simulink model "TST_TCPrt_TrqLim"  (R2016b)
settings: Solver=FixedStepDiscrete  StartTime=0.0  StopTime=simTime  FixedStep=sampleTime  RelTol=1e-3
values from neighbouring files (symbols this model uses):
  testCase = 1    [initTST_TCPrt_TrqLim_001.m]    (also in initTST_TCPrt_TrqLim_002.m = 2)
libraries: simulink x3
settings Model: Creator=wolf072601  LastModifiedBy=wolf072601
settings DebuggingCC: SignalRangeChecking=error

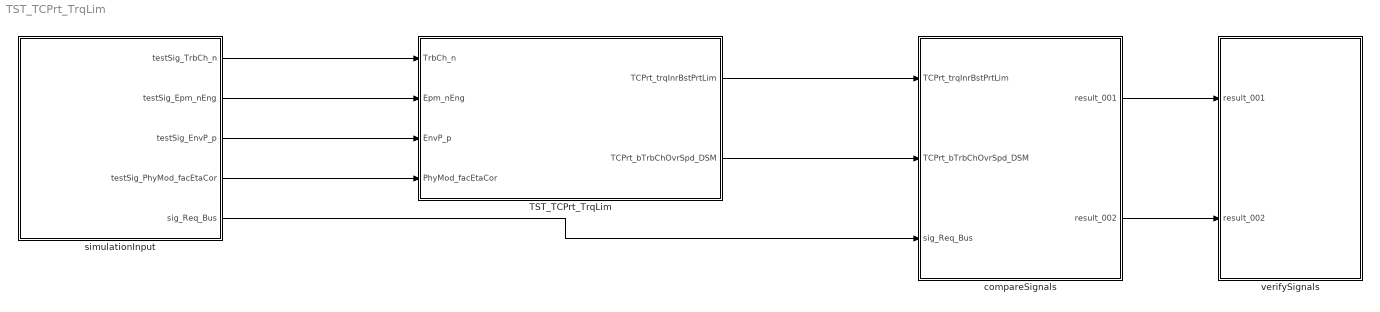
== system TST_TCPrt_TrqLim ==
  TST_TCPrt_TrqLim : Subsystem
  compareSignals : Subsystem
  simulationInput : Subsystem
  verifySignals : Subsystem
  wires:
  simulationInput/1(testSig_TrbCh_n) -> TST_TCPrt_TrqLim/1(TrbCh_n)
  simulationInput/2(testSig_Epm_nEng) -> TST_TCPrt_TrqLim/2(Epm_nEng)
  simulationInput/3(testSig_EnvP_p) -> TST_TCPrt_TrqLim/3(EnvP_p)
  simulationInput/4(testSig_PhyMod_facEtaCor) -> TST_TCPrt_TrqLim/4(PhyMod_facEtaCor)
  TST_TCPrt_TrqLim/1(TCPrt_trqInrBstPrtLim) -> compareSignals/1(TCPrt_trqInrBstPrtLim)
  TST_TCPrt_TrqLim/2(TCPrt_bTrbChOvrSpd_DSM) -> compareSignals/2(TCPrt_bTrbChOvrSpd_DSM)
  simulationInput/5(sig_Req_Bus) -> compareSignals/3(sig_Req_Bus)
  compareSignals/1(result_001) -> verifySignals/1(result_001)
  compareSignals/2(result_002) -> verifySignals/2(result_002)

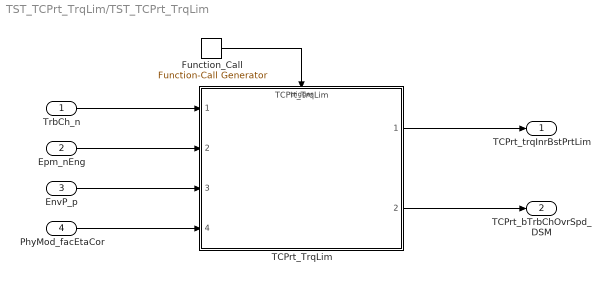
== system TST_TCPrt_TrqLim/TST_TCPrt_TrqLim ==
  TrbCh_n : Inport
  Epm_nEng : Inport  Port=2
  EnvP_p : Inport  Port=3
  PhyMod_facEtaCor : Inport  Port=4
  Function_Call : simulink/Ports & Subsystems/Function-Call Generator  sample_time=sampleTime  numberOfIterations=1
  TCPrt_TrqLim : ModelReference  ModelNameDialog=TCPrt_TrqLim  ModelReferenceVersion=1.14  TriggerPortName=function  TriggerPortTriggerType=function-call  TriggerPortStatesWhenEnabling=held
  TCPrt_trqInrBstPrtLim : Outport
  TCPrt_bTrbChOvrSpd_DSM : Outport  Port=2
  wires:
  Function_Call/1 -> TCPrt_TrqLim/Trigger
  TrbCh_n/1 -> TCPrt_TrqLim/1
  Epm_nEng/1 -> TCPrt_TrqLim/2
  EnvP_p/1 -> TCPrt_TrqLim/3
  PhyMod_facEtaCor/1 -> TCPrt_TrqLim/4
  TCPrt_TrqLim/1 -> TCPrt_trqInrBstPrtLim/1
  TCPrt_TrqLim/2 -> TCPrt_bTrbChOvrSpd_DSM/1

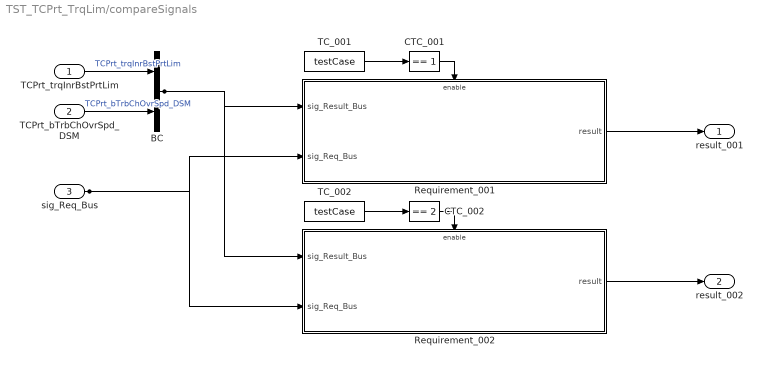
== system TST_TCPrt_TrqLim/compareSignals ==
  TCPrt_trqInrBstPrtLim : Inport
  TCPrt_bTrbChOvrSpd_DSM : Inport  Port=2
  sig_Req_Bus : Inport  Port=3
  BC : BusCreator  Inputs=2
  CTC_001 : simulink/Logic and Bit Operations/Compare To Constant  relop===  const=1  OutDataTypeStr=boolean
  CTC_002 : simulink/Logic and Bit Operations/Compare To Constant  relop===  const=2  OutDataTypeStr=boolean
  Requirement_001 : Subsystem
  Requirement_002 : Subsystem
  TC_001 : Constant  Value=testCase
  TC_002 : Constant  Value=testCase
  result_001 : Outport
  result_002 : Outport  Port=2
  wires:
  TCPrt_trqInrBstPrtLim/1 -> BC/1  "TCPrt_trqInrBstPrtLim"
  TCPrt_bTrbChOvrSpd_DSM/1 -> BC/2  "TCPrt_bTrbChOvrSpd_DSM"
  TC_001/1 -> CTC_001/1
  CTC_001/1 -> Requirement_001/Enable
  sig_Req_Bus/1 -> Requirement_001/2(sig_Req_Bus), Requirement_002/2(sig_Req_Bus)
  BC/1 -> Requirement_001/1(sig_Result_Bus), Requirement_002/1(sig_Result_Bus)
  Requirement_001/1(result) -> result_001/1
  TC_002/1 -> CTC_002/1
  CTC_002/1 -> Requirement_002/Enable
  Requirement_002/1(result) -> result_002/1

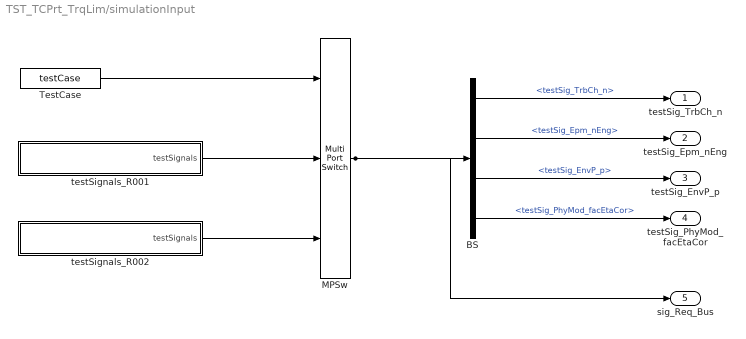
== system TST_TCPrt_TrqLim/simulationInput ==
  BS : BusSelector  OutputSignals=testSig_TrbCh_n,testSig_Epm_nEng,testSig_EnvP_p,testSig_PhyMod_facEtaCor
  MPSw : MultiPortSwitch  Inputs=2  SaturateOnIntegerOverflow=on  InputSameDT=on
  TestCase : Constant  Value=testCase
  testSignals_R001 : Subsystem
  testSignals_R002 : Subsystem
  testSig_TrbCh_n : Outport
  testSig_Epm_nEng : Outport  Port=2
  testSig_EnvP_p : Outport  Port=3
  testSig_PhyMod_facEtaCor : Outport  Port=4
  sig_Req_Bus : Outport  Port=5
  wires:
  BS/1 -> testSig_TrbCh_n/1  "<testSig_TrbCh_n>"
  BS/2 -> testSig_Epm_nEng/1  "<testSig_Epm_nEng>"
  BS/3 -> testSig_EnvP_p/1  "<testSig_EnvP_p>"
  BS/4 -> testSig_PhyMod_facEtaCor/1  "<testSig_PhyMod_facEtaCor>"
  MPSw/1 -> BS/1, sig_Req_Bus/1
  TestCase/1 -> MPSw/1
  testSignals_R001/1(testSignals) -> MPSw/2
  testSignals_R002/1(testSignals) -> MPSw/3

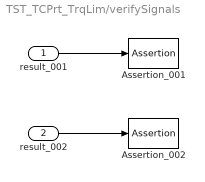
== system TST_TCPrt_TrqLim/verifySignals ==
  result_001 : Inport
  result_002 : Inport  Port=2
  Assertion_001 : Assertion  Enabled=off
  Assertion_002 : Assertion  Enabled=off
  wires:
  result_001/1 -> Assertion_001/1
  result_002/1 -> Assertion_002/1

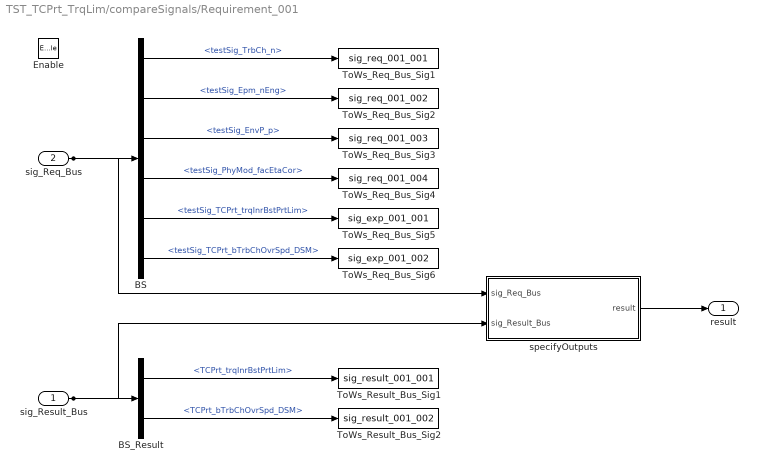
== system TST_TCPrt_TrqLim/compareSignals/Requirement_001 ==
  sig_Result_Bus : Inport
  sig_Req_Bus : Inport  Port=2
  Enable : EnablePort
  BS : BusSelector  OutputSignals=testSig_TrbCh_n,testSig_Epm_nEng,testSig_EnvP_p,testSig_PhyMod_facEtaCor,testSig_TCPrt_trqInrBstPrtLim,testSig_TCPrt_bTrbChOvrSpd_DSM
  BS_Result : BusSelector  OutputSignals=TCPrt_trqInrBstPrtLim,TCPrt_bTrbChOvrSpd_DSM
  ToWs_Req_Bus_Sig1 : ToWorkspace  VariableName=sig_req_001_001  SaveFormat=Structure With Time
  ToWs_Req_Bus_Sig2 : ToWorkspace  VariableName=sig_req_001_002  SaveFormat=Structure With Time
  ToWs_Req_Bus_Sig3 : ToWorkspace  VariableName=sig_req_001_003  SaveFormat=Structure With Time
  ToWs_Req_Bus_Sig4 : ToWorkspace  VariableName=sig_req_001_004  SaveFormat=Structure With Time
  ToWs_Req_Bus_Sig5 : ToWorkspace  VariableName=sig_exp_001_001  SaveFormat=Structure With Time
  ToWs_Req_Bus_Sig6 : ToWorkspace  VariableName=sig_exp_001_002  SaveFormat=Structure With Time
  ToWs_Result_Bus_Sig1 : ToWorkspace  VariableName=sig_result_001_001  SaveFormat=Structure With Time
  ToWs_Result_Bus_Sig2 : ToWorkspace  VariableName=sig_result_001_002  SaveFormat=Structure With Time
  specifyOutputs : Subsystem
  result : Outport
  wires:
  sig_Req_Bus/1 -> BS/1, specifyOutputs/1(sig_Req_Bus)
  BS/1 -> ToWs_Req_Bus_Sig1/1  "<testSig_TrbCh_n>"
  BS/2 -> ToWs_Req_Bus_Sig2/1  "<testSig_Epm_nEng>"
  BS/3 -> ToWs_Req_Bus_Sig3/1  "<testSig_EnvP_p>"
  BS/4 -> ToWs_Req_Bus_Sig4/1  "<testSig_PhyMod_facEtaCor>"
  BS/5 -> ToWs_Req_Bus_Sig5/1  "<testSig_TCPrt_trqInrBstPrtLim>"
  BS/6 -> ToWs_Req_Bus_Sig6/1  "<testSig_TCPrt_bTrbChOvrSpd_DSM>"
  sig_Result_Bus/1 -> BS_Result/1, specifyOutputs/2(sig_Result_Bus)
  BS_Result/1 -> ToWs_Result_Bus_Sig1/1  "<TCPrt_trqInrBstPrtLim>"
  BS_Result/2 -> ToWs_Result_Bus_Sig2/1  "<TCPrt_bTrbChOvrSpd_DSM>"
  specifyOutputs/1(result) -> result/1

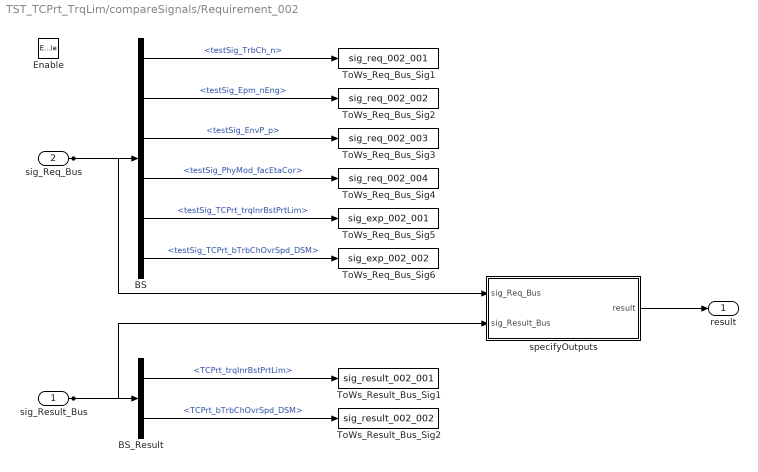
== system TST_TCPrt_TrqLim/compareSignals/Requirement_002 ==
  sig_Result_Bus : Inport
  sig_Req_Bus : Inport  Port=2
  Enable : EnablePort
  BS : BusSelector  OutputSignals=testSig_TrbCh_n,testSig_Epm_nEng,testSig_EnvP_p,testSig_PhyMod_facEtaCor,testSig_TCPrt_trqInrBstPrtLim,testSig_TCPrt_bTrbChOvrSpd_DSM
  BS_Result : BusSelector  OutputSignals=TCPrt_trqInrBstPrtLim,TCPrt_bTrbChOvrSpd_DSM
  ToWs_Req_Bus_Sig1 : ToWorkspace  VariableName=sig_req_002_001  SaveFormat=Structure With Time
  ToWs_Req_Bus_Sig2 : ToWorkspace  VariableName=sig_req_002_002  SaveFormat=Structure With Time
  ToWs_Req_Bus_Sig3 : ToWorkspace  VariableName=sig_req_002_003  SaveFormat=Structure With Time
  ToWs_Req_Bus_Sig4 : ToWorkspace  VariableName=sig_req_002_004  SaveFormat=Structure With Time
  ToWs_Req_Bus_Sig5 : ToWorkspace  VariableName=sig_exp_002_001  SaveFormat=Structure With Time
  ToWs_Req_Bus_Sig6 : ToWorkspace  VariableName=sig_exp_002_002  SaveFormat=Structure With Time
  ToWs_Result_Bus_Sig1 : ToWorkspace  VariableName=sig_result_002_001  SaveFormat=Structure With Time
  ToWs_Result_Bus_Sig2 : ToWorkspace  VariableName=sig_result_002_002  SaveFormat=Structure With Time
  specifyOutputs : Subsystem
  result : Outport
  wires:
  sig_Req_Bus/1 -> BS/1, specifyOutputs/1(sig_Req_Bus)
  BS/1 -> ToWs_Req_Bus_Sig1/1  "<testSig_TrbCh_n>"
  BS/2 -> ToWs_Req_Bus_Sig2/1  "<testSig_Epm_nEng>"
  BS/3 -> ToWs_Req_Bus_Sig3/1  "<testSig_EnvP_p>"
  BS/4 -> ToWs_Req_Bus_Sig4/1  "<testSig_PhyMod_facEtaCor>"
  BS/5 -> ToWs_Req_Bus_Sig5/1  "<testSig_TCPrt_trqInrBstPrtLim>"
  BS/6 -> ToWs_Req_Bus_Sig6/1  "<testSig_TCPrt_bTrbChOvrSpd_DSM>"
  sig_Result_Bus/1 -> BS_Result/1, specifyOutputs/2(sig_Result_Bus)
  BS_Result/1 -> ToWs_Result_Bus_Sig1/1  "<TCPrt_trqInrBstPrtLim>"
  BS_Result/2 -> ToWs_Result_Bus_Sig2/1  "<TCPrt_bTrbChOvrSpd_DSM>"
  specifyOutputs/1(result) -> result/1

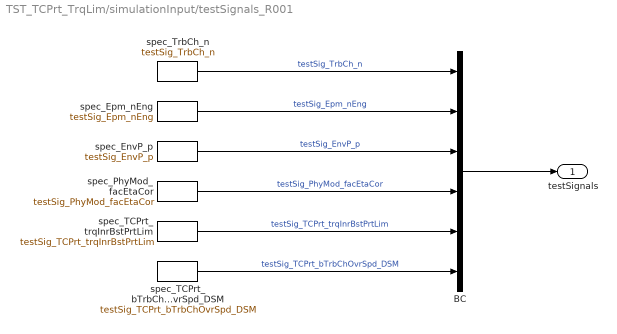
== system TST_TCPrt_TrqLim/simulationInput/testSignals_R001 ==
  BC : BusCreator  Inputs=6
  spec_EnvP_p : FromWorkspace  VariableName=testSig_EnvP_p  Interpolate=off  OutputAfterFinalValue=Holding final value
  spec_Epm_nEng : FromWorkspace  VariableName=testSig_Epm_nEng  Interpolate=off  OutputAfterFinalValue=Holding final value
  spec_PhyMod_facEtaCor : FromWorkspace  VariableName=testSig_PhyMod_facEtaCor  Interpolate=off  OutputAfterFinalValue=Holding final value
  spec_TCPrt_bTrbChOvrSpd_DSM : FromWorkspace  VariableName=testSig_TCPrt_bTrbChOvrSpd_DSM  Interpolate=off  OutputAfterFinalValue=Holding final value
  spec_TCPrt_trqInrBstPrtLim : FromWorkspace  VariableName=testSig_TCPrt_trqInrBstPrtLim  Interpolate=off  OutputAfterFinalValue=Holding final value
  spec_TrbCh_n : FromWorkspace  VariableName=testSig_TrbCh_n  Interpolate=off  OutputAfterFinalValue=Holding final value
  testSignals : Outport
  wires:
  BC/1 -> testSignals/1
  spec_TrbCh_n/1 -> BC/1  "testSig_TrbCh_n"
  spec_Epm_nEng/1 -> BC/2  "testSig_Epm_nEng"
  spec_EnvP_p/1 -> BC/3  "testSig_EnvP_p"
  spec_PhyMod_facEtaCor/1 -> BC/4  "testSig_PhyMod_facEtaCor"
  spec_TCPrt_trqInrBstPrtLim/1 -> BC/5  "testSig_TCPrt_trqInrBstPrtLim"
  spec_TCPrt_bTrbChOvrSpd_DSM/1 -> BC/6  "testSig_TCPrt_bTrbChOvrSpd_DSM"

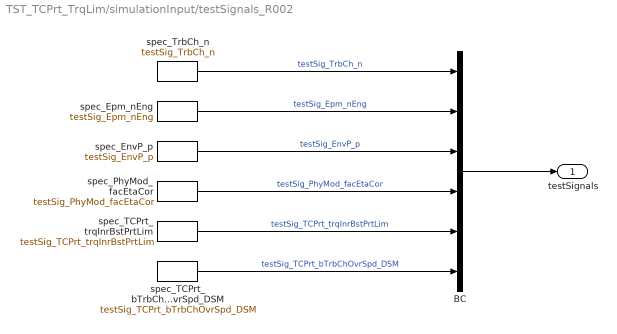
== system TST_TCPrt_TrqLim/simulationInput/testSignals_R002 ==
  BC : BusCreator  Inputs=6
  spec_EnvP_p : FromWorkspace  VariableName=testSig_EnvP_p  Interpolate=off  OutputAfterFinalValue=Holding final value
  spec_Epm_nEng : FromWorkspace  VariableName=testSig_Epm_nEng  Interpolate=off  OutputAfterFinalValue=Holding final value
  spec_PhyMod_facEtaCor : FromWorkspace  VariableName=testSig_PhyMod_facEtaCor  Interpolate=off  OutputAfterFinalValue=Holding final value
  spec_TCPrt_bTrbChOvrSpd_DSM : FromWorkspace  VariableName=testSig_TCPrt_bTrbChOvrSpd_DSM  Interpolate=off  OutputAfterFinalValue=Holding final value
  spec_TCPrt_trqInrBstPrtLim : FromWorkspace  VariableName=testSig_TCPrt_trqInrBstPrtLim  Interpolate=off  OutputAfterFinalValue=Holding final value
  spec_TrbCh_n : FromWorkspace  VariableName=testSig_TrbCh_n  Interpolate=off  OutputAfterFinalValue=Holding final value
  testSignals : Outport
  wires:
  BC/1 -> testSignals/1
  spec_TrbCh_n/1 -> BC/1  "testSig_TrbCh_n"
  spec_Epm_nEng/1 -> BC/2  "testSig_Epm_nEng"
  spec_EnvP_p/1 -> BC/3  "testSig_EnvP_p"
  spec_PhyMod_facEtaCor/1 -> BC/4  "testSig_PhyMod_facEtaCor"
  spec_TCPrt_trqInrBstPrtLim/1 -> BC/5  "testSig_TCPrt_trqInrBstPrtLim"
  spec_TCPrt_bTrbChOvrSpd_DSM/1 -> BC/6  "testSig_TCPrt_bTrbChOvrSpd_DSM"

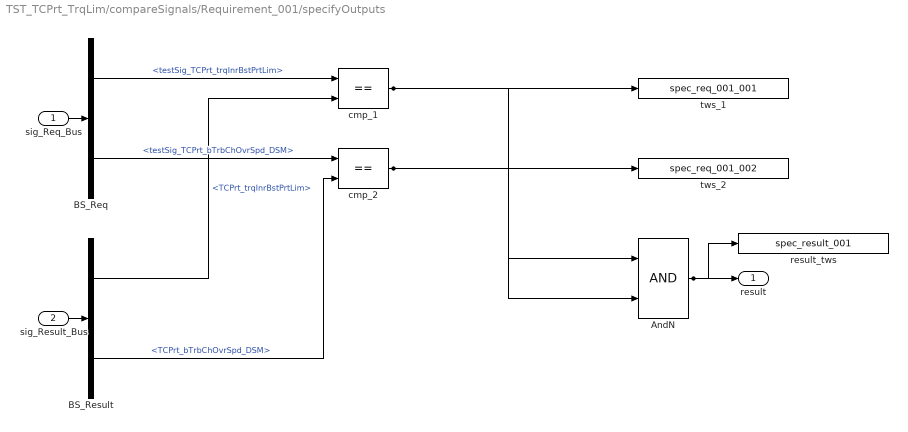
== system TST_TCPrt_TrqLim/compareSignals/Requirement_001/specifyOutputs ==
  sig_Req_Bus : Inport
  sig_Result_Bus : Inport  Port=2
  AndN : Logic
  BS_Req : BusSelector  OutputSignals=testSig_TCPrt_trqInrBstPrtLim,testSig_TCPrt_bTrbChOvrSpd_DSM
  BS_Result : BusSelector  OutputSignals=TCPrt_trqInrBstPrtLim,TCPrt_bTrbChOvrSpd_DSM
  cmp_1 : RelationalOperator  Operator===  RndMeth=Nearest  InputSameDT=on
  cmp_2 : RelationalOperator  Operator===  RndMeth=Nearest  InputSameDT=on
  result_tws : ToWorkspace  VariableName=spec_result_001
  tws_1 : ToWorkspace  VariableName=spec_req_001_001
  tws_2 : ToWorkspace  VariableName=spec_req_001_002
  result : Outport
  wires:
  sig_Req_Bus/1 -> BS_Req/1
  sig_Result_Bus/1 -> BS_Result/1
  AndN/1 -> result/1, result_tws/1
  BS_Req/1 -> cmp_1/1  "<testSig_TCPrt_trqInrBstPrtLim>"
  BS_Result/1 -> cmp_1/2  "<TCPrt_trqInrBstPrtLim>"
  cmp_1/1 -> tws_1/1, AndN/1
  BS_Req/2 -> cmp_2/1  "<testSig_TCPrt_bTrbChOvrSpd_DSM>"
  BS_Result/2 -> cmp_2/2  "<TCPrt_bTrbChOvrSpd_DSM>"
  cmp_2/1 -> tws_2/1, AndN/2

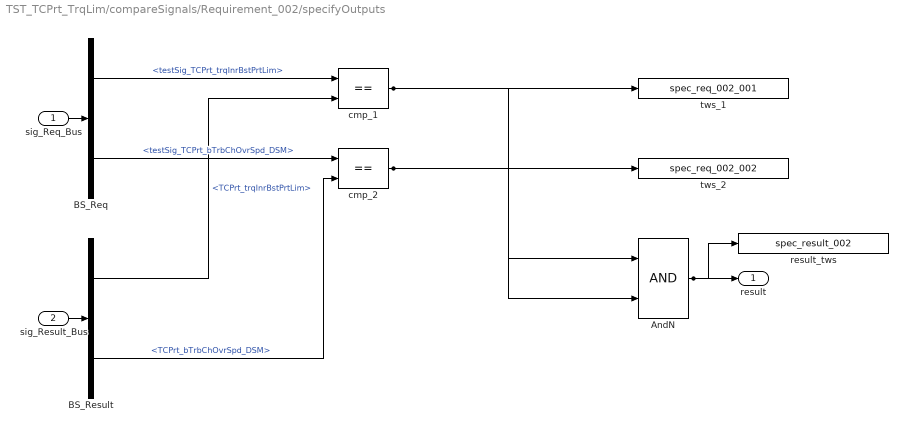
== system TST_TCPrt_TrqLim/compareSignals/Requirement_002/specifyOutputs ==
  sig_Req_Bus : Inport
  sig_Result_Bus : Inport  Port=2
  AndN : Logic
  BS_Req : BusSelector  OutputSignals=testSig_TCPrt_trqInrBstPrtLim,testSig_TCPrt_bTrbChOvrSpd_DSM
  BS_Result : BusSelector  OutputSignals=TCPrt_trqInrBstPrtLim,TCPrt_bTrbChOvrSpd_DSM
  cmp_1 : RelationalOperator  Operator===  RndMeth=Nearest  InputSameDT=on
  cmp_2 : RelationalOperator  Operator===  RndMeth=Nearest  InputSameDT=on
  result_tws : ToWorkspace  VariableName=spec_result_002
  tws_1 : ToWorkspace  VariableName=spec_req_002_001
  tws_2 : ToWorkspace  VariableName=spec_req_002_002
  result : Outport
  wires:
  sig_Req_Bus/1 -> BS_Req/1
  sig_Result_Bus/1 -> BS_Result/1
  AndN/1 -> result/1, result_tws/1
  BS_Req/1 -> cmp_1/1  "<testSig_TCPrt_trqInrBstPrtLim>"
  BS_Result/1 -> cmp_1/2  "<TCPrt_trqInrBstPrtLim>"
  cmp_1/1 -> tws_1/1, AndN/1
  BS_Req/2 -> cmp_2/1  "<testSig_TCPrt_bTrbChOvrSpd_DSM>"
  BS_Result/2 -> cmp_2/2  "<TCPrt_bTrbChOvrSpd_DSM>"
  cmp_2/1 -> tws_2/1, AndN/2
